simulink library "ADCgap_lib"  (Simulink 7.2)
settings: Solver=ode1  StartTime=0.0  StopTime=Inf  FixedStep=0.001  RelTol=1e-3
PostLoadFcn:
  | , if any(exist('dsrtsu_mdlpostloadfcn', 'file') == [2, 3, 6]), try dsrtsu_mdlpostloadfcn('Execute', bdroot); catch fprintf('Error in PostLoadFcn (dsrtsu_mdlpostloadfcn) for model "%s":\n %s\n', bdroot, lasterr); end, end,
libraries: simulink x1
settings Model: DSRTSU_INTERNAL_RTI_VER=330  DSRTSU_INTERNAL_RTI_TYPE=rti1005  Creator=gtmdev  LastModifiedBy=cbuttril

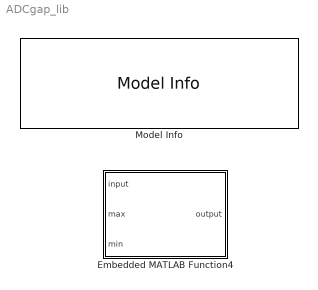
== system ADCgap_lib ==
  Embedded MATLAB Function4 : Stateflow chart
  Model Info : simulink/Model-Wide Utilities/Model Info  SystemSampleTime=-1  InitialBlockCM=None  BlockCM=None  Frame=on  DisplayStringWithTags=|  HorizontalTextAlignment=Center  LeftAlignmentValue=0.5  SourceBlockDiagram=ADCgap_lib  TagMaxNumber=20
      | ADC Gaps Library
      | %<ModelVersion>
      | Las modified by %<LastModifiedBy> on %<LastModificationDate>

== matlab function Embedded MATLAB Function4 ==
  data: input input double; output output double; max input double; min input double
function output = ADCgap(input, max, min)
% This block supports the Embedded MATLAB subset.
% See the help menu for details. 

persistent last_output;

if isempty(last_output)
    last_output = 0.0;
end

output = input;
if (input < max && input > min)
    if (last_output >= max)
        output = max;
    elseif (last_output <= min)
        output = min;
    end;
end;

last_output = output;
